simulink model "sim_new_traj_only_att_ctrl"  (R2020a)
settings: Solver=ode4  StartTime=0.0  StopTime=30.0  FixedStep=0.01  RelTol=1e-3
values from neighbouring files (symbols this model uses):
  beta_Phi_1 = pp0 * cal_frac_squ( 3, p_p0_plus_1, q_p0_plus_1 )                          * cal_frac_squ( eps_s_bar / pi, p_p0_min_2, q_p0_min_2 )                          / ( 2 * ( 2 * pp0 - 1 ) * tanh( gamma0 * ( eps_s_bar / pi ) / 2 ) )                          - ( cal_frac_squ( 3, p_p0_plus_1, q_p0_plus_1 ) * gamma0 / ( 4 * ( 2 * pp0 -1 ) ) )                          * cal_frac_squ( eps_s_bar / pi, p_p0_min_ ...(+136 chars)    [init_new_traj_only_att_ctrl.m]
  beta_Phi_2 = ( 1 - pp0 ) * cal_frac_squ( 3, p_p0_plus_1, q_p0_plus_1 )                          / ( 2 * ( 1 - 2 * pp0 ) * cal_frac_squ( eps_s_bar / pi, p_p0_0, q_p0_0 ) * tanh( gamma0 * ( eps_s_bar / pi ) / 2 ) )                          - ( cal_frac_squ( 3, p_p0_plus_1, q_p0_plus_1 ) * gamma0 / ( 4 * ( 1 - 2 * pp0 ) ) )                          * cal_frac_squ( eps_s_bar / pi, p_1_min_p0, q_1_min_p0 )          ...(+112 chars)    [init_new_traj_only_att_ctrl.m]
  c1_diff_sigma_bar_w = diag([12; 12; 12])    [init_new_traj_only_att_ctrl.m]
  c1_diff_ui = diag([25; 30; 20])    [init_new_traj_only_att_ctrl.m]
  c2_diff_sigma_bar_w = diag([12; 12; 12])    [init_new_traj_only_att_ctrl.m]
  c2_diff_ui = diag([50; 50; 10])    [init_new_traj_only_att_ctrl.m]
  c3_diff_sigma_bar_w = diag([15; 15; 15])    [init_new_traj_only_att_ctrl.m]
  c3_diff_ui = diag([15; 15; 10])    [init_new_traj_only_att_ctrl.m]
  c_w_1 = diag( [20; 15; 15] )    [init_new_traj_only_att_ctrl.m]
  c_w_2 = diag( [20; 15; 15] )    [init_new_traj_only_att_ctrl.m]
  c_w_3 = diag( [2; 2; 2] )    [init_new_traj_only_att_ctrl.m]
  cS0 = diag( [4.5; 4.5; 4.5] )    [init_new_traj_only_att_ctrl.m]
  dw_aa_t = 0.2 * ones(3, 5) + ( 1.0 - 0.2 ) * rand(3, 5)    [init_new_traj_only_att_ctrl.m]
  dw_ff_t = [ 0.4 * ones(1, 5) + ( 1.0 - 0.4 ) * rand(1, 5);                      0.4 * ones(1, 5) + ( 1.0 - 0.4 ) * rand(1, 5);                      0.2 * ones(1, 5) + ( 0.6 - 0.2 ) * rand(1, 5) ]    [init_new_traj_only_att_ctrl.m]
  dw_phi_t = ( - pi / 2 ) * ones(3, 5) + ( pi / 2 - ( - pi / 2 ) ) * rand(3, 5)    [init_new_traj_only_att_ctrl.m]
  dwci_init = zeros(3,5)    [init_new_traj_only_att_ctrl.m]
  eps_s_bar_div_pi = eps_s_bar / pi    (= 0.03)    [init_new_traj_only_att_ctrl.m]
  gamma0 = 20    [init_new_traj_only_att_ctrl.m]
  h1w = diag([20.0; 20.0; 20.0])    [init_new_traj_only_att_ctrl.m]
  h2w = diag([30.0; 35.0; 35.0])    [init_new_traj_only_att_ctrl.m]
  h3w = diag([30.0; 25.0; 30.0])    [init_new_traj_only_att_ctrl.m]
  Ji = zeros(3,3,NF)    [init_new_traj_only_att_ctrl.m]
  k_J_0 = diag( [1; 1; 1] )    [init_new_traj_only_att_ctrl.m]
  Lamd_diff_sigma_bar_w = 0.8    [init_new_traj_only_att_ctrl.m]
  Lamd_diff_ui = 0.8    [init_new_traj_only_att_ctrl.m]
  mu_c_theta = 100    [init_new_traj_only_att_ctrl.m]
  mu_d_w = 100    [init_new_traj_only_att_ctrl.m]
  pos0 = zeros(3, 1)    [init_new_traj_only_att_ctrl.m]
  pp0 = 8 / 11    (= 0.727272727273)    [init_new_traj_only_att_ctrl.m]
  PZ0 = P0(3)    [init_new_traj_only_att_ctrl.m]
  PZ1 = 10    [init_new_traj_only_att_ctrl.m]
  Qci_init = repmat([1;0;0;0],1,NF)    [init_new_traj_only_att_ctrl.m]
  R0 = 4    [init_new_traj_only_att_ctrl.m]
  R1 = 8    [init_new_traj_only_att_ctrl.m]
  Rci_init = zeros(3,3,NF)    [init_new_traj_only_att_ctrl.m]
  Ri_init = zeros(3,3,NF)    [init_new_traj_only_att_ctrl.m]
  Rx2 = 10    [init_new_traj_only_att_ctrl.m]
  Ry2 = 6    [init_new_traj_only_att_ctrl.m]
  Rz2 = 4    [init_new_traj_only_att_ctrl.m]
  T0 = 0    [init_new_traj_only_att_ctrl.m]
  T1 = tseq1    (= 10)    [init_new_traj_only_att_ctrl.m]
  T2 = tseq1 + tseq12 + tseq2    (= 30)    [init_new_traj_only_att_ctrl.m]
  thr_p_plus_1 = cal_frac_squ( 3, p_p0_plus_1, q_p0_plus_1 )    [init_new_traj_only_att_ctrl.m]
  ui_init = zeros(3,NF)    [init_new_traj_only_att_ctrl.m]
  vel0 = zeros(3, 1)    [init_new_traj_only_att_ctrl.m]
  wci_init = zeros(3,5)    [init_new_traj_only_att_ctrl.m]
  zeta_diff_sigma_bar_w = 0.3    [init_new_traj_only_att_ctrl.m]
  zeta_diff_ui = 0.05    [init_new_traj_only_att_ctrl.m]
undefined symbols (not defined in the file or in its folder): cal_frac_squ, p_2_p0, p_alfaw1, p_alfaw2, p_beta_w_1, p_beta_w_2, p_p0_min_1, p_p0_plus_1, q_2_p0, q_alfaw1, q_alfaw2, q_beta_w_1, q_beta_w_2, q_p0_min_1, q_p0_plus_1, Qei_init, Qi_init, Rei_init, V_Phi_Rei_init, wei_init, wi_init
(part 3 of 5)

== matlab function sim_new_traj_only_att_ctrl/cal differentiator d_sigma_bar_w_hat agent 3/trans to column23 ==
  data: x input; y output
function y = fcn(x)
y = x(:);

== matlab function sim_new_traj_only_att_ctrl/cal differentiator d_sigma_bar_w_hat agent 3/trans to column24 ==
  data: x input; y output
function y = fcn(x)
y = x(:);

== matlab function sim_new_traj_only_att_ctrl/cal differentiator d_sigma_bar_w_hat agent 3/trans to column25 ==
  data: x input; y output
function y = fcn(x)
y = x(:);

== matlab function sim_new_traj_only_att_ctrl/cal differentiator d_sigma_bar_w_hat agent 4/cal differentiator ==
  data: c1 input; d_sigma_bar_v_hat output; d_dsigma_bar_v_hat output; d_d2sigma_bar_v_hat output; c2 input; c3 input; chi_t input; sigma_bar_v_sig_1 input; sigma_bar_v_sig_2 input; sigma_bar_v_sig_3 input; sigma_bar_v_sig_4 input; sigma_bar_v_sig_5 input; sigma_bar_v_sig_6 input; d_sigma_bar_v_hat input; d2_sigma_bar_v_hat input
function [d_sigma_bar_v_hat, d_dsigma_bar_v_hat, d_d2sigma_bar_v_hat] = fcn(c1, c2, c3, chi_t, sigma_bar_v_sig_1, sigma_bar_v_sig_2, sigma_bar_v_sig_3, ...
                                                                                                                                                sigma_bar_v_sig_4, sigma_bar_v_sig_5, sigma_bar_v_sig_6, d_sigma_bar_v_hat, d2_sigma_bar_v_hat)
d_d2sigma_bar_v_hat = -chi_t .* c1 * sigma_bar_v_sig_1(:) - (1 - chi_t) .* c1 * sigma_bar_v_sig_2(:);
d_dsigma_bar_v_hat = -chi_t .* c2 * sigma_bar_v_sig_3(:) - (1 - chi_t) .* c2 * sigma_bar_v_sig_4(:) + d2_sigma_bar_v_hat(:);
d_sigma_bar_v_hat = -chi_t .* c3 * sigma_bar_v_sig_5(:) - (1 - chi_t) .* c3 * sigma_bar_v_sig_6(:) + d_sigma_bar_v_hat(:);

== matlab function sim_new_traj_only_att_ctrl/cal differentiator d_sigma_bar_w_hat agent 4/cal sig ==
  data: x input; z output; y input
function z = fcn(x, y)
z = x(:) .* sign(y(:));

== matlab function sim_new_traj_only_att_ctrl/cal differentiator d_sigma_bar_w_hat agent 4/cal sig1 ==
  data: x input; z output; y input
function z = fcn(x, y)
z = x(:) .* sign(y(:));

== matlab function sim_new_traj_only_att_ctrl/cal differentiator d_sigma_bar_w_hat agent 4/cal sig2 ==
  data: x input; z output; y input
function z = fcn(x, y)
z = x(:) .* sign(y(:));

== matlab function sim_new_traj_only_att_ctrl/cal differentiator d_sigma_bar_w_hat agent 4/cal sig3 ==
  data: x input; z output; y input
function z = fcn(x, y)
z = x(:) .* sign(y(:));

== matlab function sim_new_traj_only_att_ctrl/Qei dynam agent 5 ==
  data: Qei_vec input; dQei_5 output; wei_vec input
function dQei_5 = fcn(Qei_vec, wei_vec)
%%%% 更新四元数误差微分方程
iiuav = 5;

wei = wei_vec(:,iiuav);
thetaei = Qei_vec(1,iiuav);
qei = Qei_vec(2:4,iiuav);

GammaQei = zeros(4,3);
GammaQei(1,:) = -(qei');
GammaQei(2:4,:) = thetaei*eye(3,3) + cal_askew_mat(qei);
dQei_5 = (1/2)*GammaQei*wei;

end

== matlab function sim_new_traj_only_att_ctrl/cal differentiator d_sigma_bar_w_hat agent 4/cal sig4 ==
  data: x input; z output; y input
function z = fcn(x, y)
z = x(:) .* sign(y(:));

== matlab function sim_new_traj_only_att_ctrl/cal differentiator d_sigma_bar_w_hat agent 4/cal sig5 ==
  data: x input; z output; y input
function z = fcn(x, y)
z = x(:) .* sign(y(:));

== matlab function sim_new_traj_only_att_ctrl/cal differentiator d_sigma_bar_w_hat agent 4/choose sigma_bar_w ==
  data: x input; y output
function y = fcn(x)
iiuav = 4;
y = x(:,iiuav);

== matlab function sim_new_traj_only_att_ctrl/cal differentiator d_sigma_bar_w_hat agent 4/trans to column20 ==
  data: x input; y output
function y = fcn(x)
y = x(:);

== matlab function sim_new_traj_only_att_ctrl/cal differentiator d_sigma_bar_w_hat agent 4/trans to column21 ==
  data: x input; y output
function y = fcn(x)
y = x(:);

== matlab function sim_new_traj_only_att_ctrl/cal differentiator d_sigma_bar_w_hat agent 4/trans to column22 ==
  data: x input; y output
function y = fcn(x)
y = x(:);

== matlab function sim_new_traj_only_att_ctrl/cal differentiator d_sigma_bar_w_hat agent 4/trans to column23 ==
  data: x input; y output
function y = fcn(x)
y = x(:);

== matlab function sim_new_traj_only_att_ctrl/cal differentiator d_sigma_bar_w_hat agent 4/trans to column24 ==
  data: x input; y output
function y = fcn(x)
y = x(:);

== matlab function sim_new_traj_only_att_ctrl/cal differentiator d_sigma_bar_w_hat agent 4/trans to column25 ==
  data: x input; y output
function y = fcn(x)
y = x(:);

== matlab function sim_new_traj_only_att_ctrl/cal differentiator d_sigma_bar_w_hat agent 5/cal differentiator ==
  data: c1 input; d_sigma_bar_v_hat output; d_dsigma_bar_v_hat output; d_d2sigma_bar_v_hat output; c2 input; c3 input; chi_t input; sigma_bar_v_sig_1 input; sigma_bar_v_sig_2 input; sigma_bar_v_sig_3 input; sigma_bar_v_sig_4 input; sigma_bar_v_sig_5 input; sigma_bar_v_sig_6 input; d_sigma_bar_v_hat input; d2_sigma_bar_v_hat input
function [d_sigma_bar_v_hat, d_dsigma_bar_v_hat, d_d2sigma_bar_v_hat] = fcn(c1, c2, c3, chi_t, sigma_bar_v_sig_1, sigma_bar_v_sig_2, sigma_bar_v_sig_3, ...
                                                                                                                                                sigma_bar_v_sig_4, sigma_bar_v_sig_5, sigma_bar_v_sig_6, d_sigma_bar_v_hat, d2_sigma_bar_v_hat)
d_d2sigma_bar_v_hat = -chi_t .* c1 * sigma_bar_v_sig_1(:) - (1 - chi_t) .* c1 * sigma_bar_v_sig_2(:);
d_dsigma_bar_v_hat = -chi_t .* c2 * sigma_bar_v_sig_3(:) - (1 - chi_t) .* c2 * sigma_bar_v_sig_4(:) + d2_sigma_bar_v_hat(:);
d_sigma_bar_v_hat = -chi_t .* c3 * sigma_bar_v_sig_5(:) - (1 - chi_t) .* c3 * sigma_bar_v_sig_6(:) + d_sigma_bar_v_hat(:);

== matlab function sim_new_traj_only_att_ctrl/Qi dynam agent 1 ==
  data: Qi_vec input; dQi_1 output; wi_vec input
function dQi_1 = fcn(Qi_vec, wi_vec)
%%%% 更新四元数微分方程
iiuav = 1;

wi = wi_vec(:,iiuav);
thetai = Qi_vec(1,iiuav);
qi = Qi_vec(2:4,iiuav);

GammaQi = zeros(4,3);
GammaQi(1,:) = -(qi');
GammaQi(2:4,:) = thetai*eye(3,3) + cal_askew_mat(qi);
dQi_1 = (1/2)*GammaQi*wi;

end

== matlab function sim_new_traj_only_att_ctrl/cal differentiator d_sigma_bar_w_hat agent 5/cal sig ==
  data: x input; z output; y input
function z = fcn(x, y)
z = x(:) .* sign(y(:));

== matlab function sim_new_traj_only_att_ctrl/cal differentiator d_sigma_bar_w_hat agent 5/cal sig1 ==
  data: x input; z output; y input
function z = fcn(x, y)
z = x(:) .* sign(y(:));

== matlab function sim_new_traj_only_att_ctrl/cal differentiator d_sigma_bar_w_hat agent 5/cal sig2 ==
  data: x input; z output; y input
function z = fcn(x, y)
z = x(:) .* sign(y(:));

== matlab function sim_new_traj_only_att_ctrl/cal differentiator d_sigma_bar_w_hat agent 5/cal sig3 ==
  data: x input; z output; y input
function z = fcn(x, y)
z = x(:) .* sign(y(:));

== matlab function sim_new_traj_only_att_ctrl/cal differentiator d_sigma_bar_w_hat agent 5/cal sig4 ==
  data: x input; z output; y input
function z = fcn(x, y)
z = x(:) .* sign(y(:));

== matlab function sim_new_traj_only_att_ctrl/cal differentiator d_sigma_bar_w_hat agent 5/cal sig5 ==
  data: x input; z output; y input
function z = fcn(x, y)
z = x(:) .* sign(y(:));

== matlab function sim_new_traj_only_att_ctrl/cal differentiator d_sigma_bar_w_hat agent 5/choose sigma_bar_w ==
  data: x input; y output
function y = fcn(x)
iiuav = 5;
y = x(:,iiuav);

== matlab function sim_new_traj_only_att_ctrl/cal differentiator d_sigma_bar_w_hat agent 5/trans to column20 ==
  data: x input; y output
function y = fcn(x)
y = x(:);

== matlab function sim_new_traj_only_att_ctrl/cal differentiator d_sigma_bar_w_hat agent 5/trans to column21 ==
  data: x input; y output
function y = fcn(x)
y = x(:);

== matlab function sim_new_traj_only_att_ctrl/cal differentiator d_sigma_bar_w_hat agent 5/trans to column22 ==
  data: x input; y output
function y = fcn(x)
y = x(:);

== matlab function sim_new_traj_only_att_ctrl/Qi dynam agent 2 ==
  data: Qi_vec input; dQi_2 output; wi_vec input
function dQi_2 = fcn(Qi_vec, wi_vec)
%%%% 更新四元数微分方程
iiuav = 2;

wi = wi_vec(:,iiuav);
thetai = Qi_vec(1,iiuav);
qi = Qi_vec(2:4,iiuav);

GammaQi = zeros(4,3);
GammaQi(1,:) = -(qi');
GammaQi(2:4,:) = thetai*eye(3,3) + cal_askew_mat(qi);
dQi_2 = (1/2)*GammaQi*wi;

end

== matlab function sim_new_traj_only_att_ctrl/cal differentiator d_sigma_bar_w_hat agent 5/trans to column23 ==
  data: x input; y output
function y = fcn(x)
y = x(:);

== matlab function sim_new_traj_only_att_ctrl/cal differentiator d_sigma_bar_w_hat agent 5/trans to column24 ==
  data: x input; y output
function y = fcn(x)
y = x(:);

== matlab function sim_new_traj_only_att_ctrl/cal differentiator d_sigma_bar_w_hat agent 5/trans to column25 ==
  data: x input; y output
function y = fcn(x)
y = x(:);

== matlab function sim_new_traj_only_att_ctrl/cal divide pi ==
  data: x input; y output
function y = fcn(x)
y = x ./ pi;

== matlab function sim_new_traj_only_att_ctrl/cal dw_hat agent 1 ==
  data: h3w input; Ji input; d_sigma_bar_w_vec input; sigma_bar_w_hat_vec input; dw_hat_1 output
function dw_hat_1 = fcn(h3w, Ji, d_sigma_bar_w_vec, sigma_bar_w_hat_vec)
%%%% 计算扰动观测值dw_hat
iiuav = 1;
dw_hat_1 = Ji(:,:,iiuav) * d_sigma_bar_w_vec(:,iiuav) + h3w * sigma_bar_w_hat_vec(:,iiuav);

== matlab function sim_new_traj_only_att_ctrl/cal dw_hat agent 2 ==
  data: h3w input; Ji input; d_sigma_bar_w_vec input; sigma_bar_w_hat_vec input; dw_hat_2 output
function dw_hat_2 = fcn(h3w, Ji, d_sigma_bar_w_vec, sigma_bar_w_hat_vec)
%%%% 计算扰动观测值dw_hat
iiuav = 2;
dw_hat_2 = Ji(:,:,iiuav) * d_sigma_bar_w_vec(:,iiuav) + h3w * sigma_bar_w_hat_vec(:,iiuav);

== matlab function sim_new_traj_only_att_ctrl/cal dw_hat agent 3 ==
  data: h3w input; Ji input; d_sigma_bar_w_vec input; sigma_bar_w_hat_vec input; dw_hat_3 output
function dw_hat_3 = fcn(h3w, Ji, d_sigma_bar_w_vec, sigma_bar_w_hat_vec)
%%%% 计算扰动观测值dw_hat
iiuav = 3;
dw_hat_3 = Ji(:,:,iiuav) * d_sigma_bar_w_vec(:,iiuav) + h3w * sigma_bar_w_hat_vec(:,iiuav);

== matlab function sim_new_traj_only_att_ctrl/cal dw_hat agent 4 ==
  data: h3w input; Ji input; d_sigma_bar_w_vec input; sigma_bar_w_hat_vec input; dw_hat_4 output
function dw_hat_4 = fcn(h3w, Ji, d_sigma_bar_w_vec, sigma_bar_w_hat_vec)
%%%% 计算扰动观测值dw_hat
iiuav = 4;
dw_hat_4 = Ji(:,:,iiuav) * d_sigma_bar_w_vec(:,iiuav) + h3w * sigma_bar_w_hat_vec(:,iiuav);

== matlab function sim_new_traj_only_att_ctrl/cal dw_hat agent 5 ==
  data: h3w input; Ji input; d_sigma_bar_w_vec input; sigma_bar_w_hat_vec input; dw_hat_5 output
function dw_hat_5 = fcn(h3w, Ji, d_sigma_bar_w_vec, sigma_bar_w_hat_vec)
%%%% 计算扰动观测值dw_hat
iiuav = 5;
dw_hat_5 = Ji(:,:,iiuav) * d_sigma_bar_w_vec(:,iiuav) + h3w * sigma_bar_w_hat_vec(:,iiuav);

== matlab function sim_new_traj_only_att_ctrl/Qi dynam agent 3 ==
  data: Qi_vec input; dQi_3 output; wi_vec input
function dQi_3 = fcn(Qi_vec, wi_vec)
%%%% 更新四元数微分方程
iiuav = 3;

wi = wi_vec(:,iiuav);
thetai = Qi_vec(1,iiuav);
qi = Qi_vec(2:4,iiuav);

GammaQi = zeros(4,3);
GammaQi(1,:) = -(qi');
GammaQi(2:4,:) = thetai*eye(3,3) + cal_askew_mat(qi);
dQi_3 = (1/2)*GammaQi*wi;

end

== matlab function sim_new_traj_only_att_ctrl/cal error dw_tilt ==
  data: dw_vec input; dw_hat_vec input; dw_tilt_vec output
function dw_tilt_vec = fcn(dw_vec, dw_hat_vec)
%%%% 计算扰动观测误差dw_tilt
dw_tilt_vec = zeros(3,5);
for iiuav = 1:5
    dw_tilt_vec(:,iiuav) = dw_vec(:,iiuav) - dw_hat_vec(:,iiuav);
end

== matlab function sim_new_traj_only_att_ctrl/cal sig ==
  data: x input; z output; y input
function z = fcn(x, y)
z = x(:) .* sign(y(:));

== matlab function sim_new_traj_only_att_ctrl/cal sig1 ==
  data: x input; z output; y input
function z = fcn(x, y)
z = x(:) .* sign(y(:));

== matlab function sim_new_traj_only_att_ctrl/cal sig10 ==
  data: x input; z output; y input
function z = fcn(x, y)
z = x(:) .* sign(y(:));

== matlab function sim_new_traj_only_att_ctrl/cal sig11 ==
  data: x input; z output; y input
function z = fcn(x, y)
z = x(:) .* sign(y(:));

== matlab function sim_new_traj_only_att_ctrl/cal sig12 ==
  data: x input; z output; y input
function z = fcn(x, y)
z = x(:) .* sign(y(:));

== matlab function sim_new_traj_only_att_ctrl/cal sig13 ==
  data: x input; z output; y input
function z = fcn(x, y)
z = x(:) .* sign(y(:));

== matlab function sim_new_traj_only_att_ctrl/cal sig14 ==
  data: x input; z output; y input
function z = fcn(x, y)
z = x(:) .* sign(y(:));

== matlab function sim_new_traj_only_att_ctrl/cal sig15 ==
  data: x input; z output; y input
function z = fcn(x, y)
z = x(:) .* sign(y(:));

== matlab function sim_new_traj_only_att_ctrl/cal sig16 ==
  data: x input; z output; y input
function z = fcn(x, y)
z = x(:) .* sign(y(:));

== matlab function sim_new_traj_only_att_ctrl/Qi dynam agent 4 ==
  data: Qi_vec input; dQi_4 output; wi_vec input
function dQi_4 = fcn(Qi_vec, wi_vec)
%%%% 更新四元数微分方程
iiuav = 4;

wi = wi_vec(:,iiuav);
thetai = Qi_vec(1,iiuav);
qi = Qi_vec(2:4,iiuav);

GammaQi = zeros(4,3);
GammaQi(1,:) = -(qi');
GammaQi(2:4,:) = thetai*eye(3,3) + cal_askew_mat(qi);
dQi_4 = (1/2)*GammaQi*wi;

end

== matlab function sim_new_traj_only_att_ctrl/cal sig17 ==
  data: x input; z output; y input
function z = fcn(x, y)
z = x(:) .* sign(y(:));

== matlab function sim_new_traj_only_att_ctrl/cal sig18 ==
  data: x input; z output; y input
function z = fcn(x, y)
z = x(:) .* sign(y(:));

== matlab function sim_new_traj_only_att_ctrl/cal sig19 ==
  data: x input; z output; y input
function z = fcn(x, y)
z = x(:) .* sign(y(:));

== matlab function sim_new_traj_only_att_ctrl/cal sig2 ==
  data: x input; z output; y input
function z = fcn(x, y)
z = x(:) .* sign(y(:));

== matlab function sim_new_traj_only_att_ctrl/cal sig20 ==
  data: x input; z output; y input
function z = fcn(x, y)
z = x(:) .* sign(y(:));

== matlab function sim_new_traj_only_att_ctrl/cal sig21 ==
  data: x input; z output; y input
function z = fcn(x, y)
z = x(:) .* sign(y(:));

== matlab function sim_new_traj_only_att_ctrl/cal sig22 ==
  data: x input; z output; y input
function z = fcn(x, y)
z = x(:) .* sign(y(:));

== matlab function sim_new_traj_only_att_ctrl/cal sig23 ==
  data: x input; z output; y input
function z = fcn(x, y)
z = x(:) .* sign(y(:));

== matlab function sim_new_traj_only_att_ctrl/cal sig24 ==
  data: x input; z output; y input
function z = fcn(x, y)
z = x(:) .* sign(y(:));

== matlab function sim_new_traj_only_att_ctrl/cal sig25 ==
  data: x input; z output; y input
function z = fcn(x, y)
z = x(:) .* sign(y(:));

== matlab function sim_new_traj_only_att_ctrl/Qi dynam agent 5 ==
  data: Qi_vec input; dQi_5 output; wi_vec input
function dQi_5 = fcn(Qi_vec, wi_vec)
%%%% 更新四元数微分方程
iiuav = 5;

wi = wi_vec(:,iiuav);
thetai = Qi_vec(1,iiuav);
qi = Qi_vec(2:4,iiuav);

GammaQi = zeros(4,3);
GammaQi(1,:) = -(qi');
GammaQi(2:4,:) = thetai*eye(3,3) + cal_askew_mat(qi);
dQi_5 = (1/2)*GammaQi*wi;

end

== matlab function sim_new_traj_only_att_ctrl/cal sig26 ==
  data: x input; z output; y input
function z = fcn(x, y)
z = x(:) .* sign(y(:));

== matlab function sim_new_traj_only_att_ctrl/cal sig27 ==
  data: x input; z output; y input
function z = fcn(x, y)
z = x(:) .* sign(y(:));

== matlab function sim_new_traj_only_att_ctrl/cal sig28 ==
  data: x input; z output; y input
function z = fcn(x, y)
z = x(:) .* sign(y(:));

== matlab function sim_new_traj_only_att_ctrl/cal sig29 ==
  data: x input; z output; y input
function z = fcn(x, y)
z = x(:) .* sign(y(:));

== matlab function sim_new_traj_only_att_ctrl/cal sig3 ==
  data: x input; z output; y input
function z = fcn(x, y)
z = x(:) .* sign(y(:));

== matlab function sim_new_traj_only_att_ctrl/cal sig4 ==
  data: x input; z output; y input
function z = fcn(x, y)
z = x(:) .* sign(y(:));

== matlab function sim_new_traj_only_att_ctrl/cal sig5 ==
  data: x input; z output; y input
function z = fcn(x, y)
z = x(:) .* sign(y(:));

== matlab function sim_new_traj_only_att_ctrl/cal sig6 ==
  data: x input; z output; y input
function z = fcn(x, y)
z = x(:) .* sign(y(:));

== matlab function sim_new_traj_only_att_ctrl/cal sig7 ==
  data: x input; z output; y input
function z = fcn(x, y)
z = x(:) .* sign(y(:));

== matlab function sim_new_traj_only_att_ctrl/cal sig8 ==
  data: x input; z output; y input
function z = fcn(x, y)
z = x(:) .* sign(y(:));

== matlab function sim_new_traj_only_att_ctrl/cal Fi_S agent 1 ==
  data: cS0 input; Ji input; wi_vec input; wci_vec input; wei_vec input; Fi_S_1 output; dwci_vec input; Rei_vec input; Phi_bar_psi_e_vec input
function Fi_S_1 = fcn(cS0, Ji, wi_vec, wci_vec, wei_vec, dwci_vec, Rei_vec, Phi_bar_psi_e_vec)
%%%% 计算补偿项
iiuav = 1;
Fi_S_1 = -cal_askew_mat( wi_vec(:,iiuav) ) * Ji(:,:,iiuav) * wi_vec(:,iiuav) ...
                + Ji(:,:,iiuav) * cal_askew_mat( wei_vec(:,iiuav) ) * ( Rei_vec(:,:,iiuav)' ) * wci_vec(:,iiuav) ...
                - Ji(:,:,iiuav) * ( Rei_vec(:,:,iiuav)' ) * dwci_vec(:,iiuav) ...
                + cS0 * Ji(:,:,iiuav) * Phi_bar_psi_e_vec(:,iiuav);

== matlab function sim_new_traj_only_att_ctrl/cal sig9 ==
  data: x input; z output; y input
function z = fcn(x, y)
z = x(:) .* sign(y(:));

== matlab function sim_new_traj_only_att_ctrl/cal sigma_bar_w_hat agent 1 ==
  data: h1w input; h2w input; theta_sigma_bar_w_tilt_1_vec input; d_sigma_bar_w_hat_1 output; theta_sigma_bar_w_tilt_2_vec input; d_sigma_bar_w_vec input
function d_sigma_bar_w_hat_1 = fcn(h1w, h2w, theta_sigma_bar_w_tilt_1_vec, theta_sigma_bar_w_tilt_2_vec, d_sigma_bar_w_vec)
%%%% 计算扰动观测器中虚拟速度控制量观测值sigma_w_hat的微分方程
iiuav = 1;
d_sigma_bar_w_hat_1 = d_sigma_bar_w_vec(:,iiuav) + ...
                                            h1w * theta_sigma_bar_w_tilt_1_vec(:,iiuav) + ...
                                            h2w * theta_sigma_bar_w_tilt_2_vec(:,iiuav);

== matlab function sim_new_traj_only_att_ctrl/cal sigma_bar_w_hat agent 2 ==
  data: h1w input; h2w input; theta_sigma_bar_w_tilt_1_vec input; d_sigma_bar_w_hat_2 output; theta_sigma_bar_w_tilt_2_vec input; d_sigma_bar_w_vec input
function d_sigma_bar_w_hat_2 = fcn(h1w, h2w, theta_sigma_bar_w_tilt_1_vec, theta_sigma_bar_w_tilt_2_vec, d_sigma_bar_w_vec)
%%%% 计算扰动观测器中虚拟速度控制量观测值sigma_v_hat的微分方程
iiuav = 2;
d_sigma_bar_w_hat_2 = d_sigma_bar_w_vec(:,iiuav) + ...
                                            h1w * theta_sigma_bar_w_tilt_1_vec(:,iiuav) + ...
                                            h2w * theta_sigma_bar_w_tilt_2_vec(:,iiuav);

== matlab function sim_new_traj_only_att_ctrl/cal sigma_bar_w_hat agent 3 ==
  data: h1w input; h2w input; theta_sigma_bar_w_tilt_1_vec input; d_sigma_bar_w_hat_3 output; theta_sigma_bar_w_tilt_2_vec input; d_sigma_bar_w_vec input
function d_sigma_bar_w_hat_3 = fcn(h1w, h2w, theta_sigma_bar_w_tilt_1_vec, theta_sigma_bar_w_tilt_2_vec, d_sigma_bar_w_vec)
%%%% 计算扰动观测器中虚拟速度控制量观测值sigma_w_hat的微分方程
iiuav = 3;
d_sigma_bar_w_hat_3 = d_sigma_bar_w_vec(:,iiuav) + ...
                                            h1w * theta_sigma_bar_w_tilt_1_vec(:,iiuav) + ...
                                            h2w * theta_sigma_bar_w_tilt_2_vec(:,iiuav);

== matlab function sim_new_traj_only_att_ctrl/cal sigma_bar_w_hat agent 4 ==
  data: h1w input; h2w input; theta_sigma_bar_w_tilt_1_vec input; d_sigma_bar_w_hat_4 output; theta_sigma_bar_w_tilt_2_vec input; d_sigma_bar_w_vec input
function d_sigma_bar_w_hat_4 = fcn(h1w, h2w, theta_sigma_bar_w_tilt_1_vec, theta_sigma_bar_w_tilt_2_vec, d_sigma_bar_w_vec)
%%%% 计算扰动观测器中虚拟速度控制量观测值sigma_w_hat的微分方程
iiuav = 4;
d_sigma_bar_w_hat_4 = d_sigma_bar_w_vec(:,iiuav) + ...
                                            h1w * theta_sigma_bar_w_tilt_1_vec(:,iiuav) + ...
                                            h2w * theta_sigma_bar_w_tilt_2_vec(:,iiuav);

== matlab function sim_new_traj_only_att_ctrl/cal sigma_bar_w_hat agent 5 ==
  data: h1w input; h2w input; theta_sigma_bar_w_tilt_1_vec input; d_sigma_bar_w_hat_5 output; theta_sigma_bar_w_tilt_2_vec input; d_sigma_bar_w_vec input
function d_sigma_bar_w_hat_5 = fcn(h1w, h2w, theta_sigma_bar_w_tilt_1_vec, theta_sigma_bar_w_tilt_2_vec, d_sigma_bar_w_vec)
%%%% 计算扰动观测器中虚拟速度控制量观测值sigma_w_hat的微分方程
iiuav = 5;
d_sigma_bar_w_hat_5 = d_sigma_bar_w_vec(:,iiuav) + ...
                                            h1w * theta_sigma_bar_w_tilt_1_vec(:,iiuav) + ...
                                            h2w * theta_sigma_bar_w_tilt_2_vec(:,iiuav);

== matlab function sim_new_traj_only_att_ctrl/cal sigma_w_bar ==
  data: sigma_bar_w_vec output; wi_vec input; sigma_w_vec input
function sigma_bar_w_vec = fcn(wi_vec, sigma_w_vec)
%%%% 计算姿态角速率跟踪误差
sigma_bar_w_vec = zeros(3,5);
for iiuav = 1:5
    sigma_bar_w_vec(:,iiuav) = wi_vec(:,iiuav) - sigma_w_vec(:,iiuav);
end

== matlab function sim_new_traj_only_att_ctrl/cal taui agent 1 ==
  data: c_w_1 input; c_w_2 input; c_w_3 input; k_J_0 input; tau_1 output; Ji input; Si_vec input; dw_hat_vec input; Fi_S_vec input; theta_Si_beta_w_1_vec input; theta_Si_beta_w_2_vec input
function tau_1 = fcn(c_w_1, c_w_2, c_w_3, k_J_0, Ji, Si_vec, dw_hat_vec, ...
                                        Fi_S_vec, theta_Si_beta_w_1_vec, theta_Si_beta_w_2_vec)
%%%% 计算用于姿态控制的驱动力矩控制输入
iiuav = 1;
tau_1 = -c_w_1 * theta_Si_beta_w_1_vec(:,iiuav) - c_w_2 * theta_Si_beta_w_2_vec(:,iiuav) - c_w_3 * Si_vec(:,iiuav) ...
                - dw_hat_vec(:,iiuav) - k_J_0 * inv( Ji(:,:,iiuav) ) * Fi_S_vec(:,iiuav);
end

== matlab function sim_new_traj_only_att_ctrl/cal taui agent 2 ==
  data: c_w_1 input; c_w_2 input; c_w_3 input; k_J_0 input; tau_2 output; Ji input; Si_vec input; dw_hat_vec input; Fi_S_vec input; theta_Si_beta_w_1_vec input; theta_Si_beta_w_2_vec input
function tau_2 = fcn(c_w_1, c_w_2, c_w_3, k_J_0, Ji, Si_vec, dw_hat_vec, ...
                                        Fi_S_vec, theta_Si_beta_w_1_vec, theta_Si_beta_w_2_vec)
%%%% 计算用于姿态控制的驱动力矩控制输入
iiuav = 2;
tau_2 = -c_w_1 * theta_Si_beta_w_1_vec(:,iiuav) - c_w_2 * theta_Si_beta_w_2_vec(:,iiuav) - c_w_3 * Si_vec(:,iiuav) ...
                - dw_hat_vec(:,iiuav) - k_J_0 * inv( Ji(:,:,iiuav) ) * Fi_S_vec(:,iiuav);
end

== matlab function sim_new_traj_only_att_ctrl/cal taui agent 3 ==
  data: c_w_1 input; c_w_2 input; c_w_3 input; k_J_0 input; tau_3 output; Ji input; Si_vec input; dw_hat_vec input; Fi_S_vec input; theta_Si_beta_w_1_vec input; theta_Si_beta_w_2_vec input
function tau_3 = fcn(c_w_1, c_w_2, c_w_3, k_J_0, Ji, Si_vec, dw_hat_vec, ...
                                        Fi_S_vec, theta_Si_beta_w_1_vec, theta_Si_beta_w_2_vec)
%%%% 计算用于姿态控制的驱动力矩控制输入
iiuav = 3;
tau_3 = -c_w_1 * theta_Si_beta_w_1_vec(:,iiuav) - c_w_2 * theta_Si_beta_w_2_vec(:,iiuav) - c_w_3 * Si_vec(:,iiuav) ...
                - dw_hat_vec(:,iiuav) - k_J_0 * inv( Ji(:,:,iiuav) ) * Fi_S_vec(:,iiuav);
end

== matlab function sim_new_traj_only_att_ctrl/cal taui agent 4 ==
  data: c_w_1 input; c_w_2 input; c_w_3 input; k_J_0 input; tau_4 output; Ji input; Si_vec input; dw_hat_vec input; Fi_S_vec input; theta_Si_beta_w_1_vec input; theta_Si_beta_w_2_vec input
function tau_4 = fcn(c_w_1, c_w_2, c_w_3, k_J_0, Ji, Si_vec, dw_hat_vec, ...
                                        Fi_S_vec, theta_Si_beta_w_1_vec, theta_Si_beta_w_2_vec)
%%%% 计算用于姿态控制的驱动力矩控制输入
iiuav = 4;
tau_4 = -c_w_1 * theta_Si_beta_w_1_vec(:,iiuav) - c_w_2 * theta_Si_beta_w_2_vec(:,iiuav) - c_w_3 * Si_vec(:,iiuav) ...
                - dw_hat_vec(:,iiuav) - k_J_0 * inv( Ji(:,:,iiuav) ) * Fi_S_vec(:,iiuav);
end

== matlab function sim_new_traj_only_att_ctrl/cal taui agent 5 ==
  data: c_w_1 input; c_w_2 input; c_w_3 input; k_J_0 input; tau_5 output; Ji input; Si_vec input; dw_hat_vec input; Fi_S_vec input; theta_Si_beta_w_1_vec input; theta_Si_beta_w_2_vec input
function tau_5 = fcn(c_w_1, c_w_2, c_w_3, k_J_0, Ji, Si_vec, dw_hat_vec, ...
                                        Fi_S_vec, theta_Si_beta_w_1_vec, theta_Si_beta_w_2_vec)
%%%% 计算用于姿态控制的驱动力矩控制输入
iiuav = 5;
tau_5 = -c_w_1 * theta_Si_beta_w_1_vec(:,iiuav) - c_w_2 * theta_Si_beta_w_2_vec(:,iiuav) - c_w_3 * Si_vec(:,iiuav) ...
                - dw_hat_vec(:,iiuav) - k_J_0 * inv( Ji(:,:,iiuav) ) * Fi_S_vec(:,iiuav);
end

== matlab function sim_new_traj_only_att_ctrl/cal Fi_S agent 2 ==
  data: cS0 input; Ji input; wi_vec input; wci_vec input; wei_vec input; Fi_S_2 output; dwci_vec input; Rei_vec input; Phi_bar_psi_e_vec input
function Fi_S_2 = fcn(cS0, Ji, wi_vec, wci_vec, wei_vec, dwci_vec, Rei_vec, Phi_bar_psi_e_vec)
%%%% 计算补偿项
iiuav = 2;
Fi_S_2 = -cal_askew_mat( wi_vec(:,iiuav) ) * Ji(:,:,iiuav) * wi_vec(:,iiuav) ...
                + Ji(:,:,iiuav) * cal_askew_mat( wei_vec(:,iiuav) ) * ( Rei_vec(:,:,iiuav)' ) * wci_vec(:,iiuav) ...
                - Ji(:,:,iiuav) * ( Rei_vec(:,:,iiuav)' ) * dwci_vec(:,iiuav) ...
                + cS0 * Ji(:,:,iiuav) * Phi_bar_psi_e_vec(:,iiuav);

== matlab function sim_new_traj_only_att_ctrl/cal theta_Si_beta_w agent 1 ==
  data: mu_c_theta input; Si_squ_beta_w_1_vec input; theta_Si_beta_w_1_node_1 output; Si_squ_beta_w_2_vec input; Si_vec input; theta_Si_beta_w_2_node_1 output
function [theta_Si_beta_w_1_node_1, theta_Si_beta_w_2_node_1] = fcn(mu_c_theta, Si_squ_beta_w_1_vec, Si_squ_beta_w_2_vec, Si_vec)
%%%% 计算平滑递增函数
iiuav = 1;
theta_Si_beta_w_1_node_1 = Si_squ_beta_w_1_vec(:, iiuav) .* ( -1 + 2 ./ ( 1 + exp( -mu_c_theta .* Si_vec(:,iiuav) ) ) );
theta_Si_beta_w_2_node_1 = Si_squ_beta_w_2_vec(:, iiuav) .* ( -1 + 2 ./ ( 1 + exp( -mu_c_theta .* Si_vec(:,iiuav) ) ) );

== matlab function sim_new_traj_only_att_ctrl/cal theta_Si_beta_w agent 2 ==
  data: mu_c_theta input; Si_squ_beta_w_1_vec input; theta_Si_beta_w_1_node_2 output; Si_squ_beta_w_2_vec input; Si_vec input; theta_Si_beta_w_2_node_2 output
function [theta_Si_beta_w_1_node_2, theta_Si_beta_w_2_node_2] = fcn(mu_c_theta, Si_squ_beta_w_1_vec, Si_squ_beta_w_2_vec, Si_vec)
%%%% 计算平滑递增函数
iiuav = 2;
theta_Si_beta_w_1_node_2 = Si_squ_beta_w_1_vec(:, iiuav) .* ( -1 + 2 ./ ( 1 + exp( -mu_c_theta .* Si_vec(:,iiuav) ) ) );
theta_Si_beta_w_2_node_2 = Si_squ_beta_w_2_vec(:, iiuav) .* ( -1 + 2 ./ ( 1 + exp( -mu_c_theta .* Si_vec(:,iiuav) ) ) );

== matlab function sim_new_traj_only_att_ctrl/cal theta_Si_beta_w agent 3 ==
  data: mu_c_theta input; Si_squ_beta_w_1_vec input; theta_Si_beta_w_1_node_3 output; Si_squ_beta_w_2_vec input; Si_vec input; theta_Si_beta_w_2_node_3 output
function [theta_Si_beta_w_1_node_3, theta_Si_beta_w_2_node_3] = fcn(mu_c_theta, Si_squ_beta_w_1_vec, Si_squ_beta_w_2_vec, Si_vec)
%%%% 计算平滑递增函数
iiuav = 3;
theta_Si_beta_w_1_node_3 = Si_squ_beta_w_1_vec(:, iiuav) .* ( -1 + 2 ./ ( 1 + exp( -mu_c_theta .* Si_vec(:,iiuav) ) ) );
theta_Si_beta_w_2_node_3 = Si_squ_beta_w_2_vec(:, iiuav) .* ( -1 + 2 ./ ( 1 + exp( -mu_c_theta .* Si_vec(:,iiuav) ) ) );

== matlab function sim_new_traj_only_att_ctrl/cal theta_Si_beta_w agent 4 ==
  data: mu_c_theta input; Si_squ_beta_w_1_vec input; theta_Si_beta_w_1_node_4 output; Si_squ_beta_w_2_vec input; Si_vec input; theta_Si_beta_w_2_node_4 output
function [theta_Si_beta_w_1_node_4, theta_Si_beta_w_2_node_4] = fcn(mu_c_theta, Si_squ_beta_w_1_vec, Si_squ_beta_w_2_vec, Si_vec)
%%%% 计算平滑递增函数
iiuav = 4;
theta_Si_beta_w_1_node_4 = Si_squ_beta_w_1_vec(:, iiuav) .* ( -1 + 2 ./ ( 1 + exp( -mu_c_theta .* Si_vec(:,iiuav) ) ) );
theta_Si_beta_w_2_node_4 = Si_squ_beta_w_2_vec(:, iiuav) .* ( -1 + 2 ./ ( 1 + exp( -mu_c_theta .* Si_vec(:,iiuav) ) ) );

== matlab function sim_new_traj_only_att_ctrl/cal theta_Si_beta_w agent 5 ==
  data: mu_c_theta input; Si_squ_beta_w_1_vec input; theta_Si_beta_w_1_node_5 output; Si_squ_beta_w_2_vec input; Si_vec input; theta_Si_beta_w_2_node_5 output
function [theta_Si_beta_w_1_node_5, theta_Si_beta_w_2_node_5] = fcn(mu_c_theta, Si_squ_beta_w_1_vec, Si_squ_beta_w_2_vec, Si_vec)
%%%% 计算平滑递增函数
iiuav = 5;
theta_Si_beta_w_1_node_5 = Si_squ_beta_w_1_vec(:, iiuav) .* ( -1 + 2 ./ ( 1 + exp( -mu_c_theta .* Si_vec(:,iiuav) ) ) );
theta_Si_beta_w_2_node_5 = Si_squ_beta_w_2_vec(:, iiuav) .* ( -1 + 2 ./ ( 1 + exp( -mu_c_theta .* Si_vec(:,iiuav) ) ) );

== matlab function sim_new_traj_only_att_ctrl/cal theta_sigma_bar_w_tilt agent 1 ==
  data: alfa_theta_obs_w input; sigma_bar_w_tilt_squ_1_1 input; theta_sigma_bar_w_tilt_1_1 output; sigma_bar_w_tilt_squ_2_1 input; sigma_bar_w_tilt_vec input; theta_sigma_bar_w_tilt_2_1 output
function [theta_sigma_bar_w_tilt_1_1, theta_sigma_bar_w_tilt_2_1] = fcn(alfa_theta_obs_w, sigma_bar_w_tilt_squ_1_1, sigma_bar_w_tilt_squ_2_1, sigma_bar_w_tilt_vec)
%%%% 计算平滑递增函数
iiuav = 1;
theta_sigma_bar_w_tilt_1_1 = sigma_bar_w_tilt_squ_1_1(:) .* ( -1 + 2 ./ ( 1 + exp( -alfa_theta_obs_w .* sigma_bar_w_tilt_vec(:,iiuav) ) ) );
theta_sigma_bar_w_tilt_2_1 = sigma_bar_w_tilt_squ_2_1(:) .* ( -1 + 2 ./ ( 1 + exp( -alfa_theta_obs_w .* sigma_bar_w_tilt_vec(:,iiuav) ) ) );

== matlab function sim_new_traj_only_att_ctrl/cal theta_sigma_bar_w_tilt agent 2 ==
  data: alfa_theta_obs_w input; sigma_bar_w_tilt_squ_1_2 input; theta_sigma_bar_w_tilt_1_2 output; sigma_bar_w_tilt_squ_2_2 input; sigma_bar_w_tilt_vec input; theta_sigma_bar_w_tilt_2_2 output
function [theta_sigma_bar_w_tilt_1_2, theta_sigma_bar_w_tilt_2_2] = fcn(alfa_theta_obs_w, sigma_bar_w_tilt_squ_1_2, sigma_bar_w_tilt_squ_2_2, sigma_bar_w_tilt_vec)
%%%% 计算平滑递增函数
iiuav = 2;
theta_sigma_bar_w_tilt_1_2 = sigma_bar_w_tilt_squ_1_2(:) .* ( -1 + 2 ./ ( 1 + exp( -alfa_theta_obs_w .* sigma_bar_w_tilt_vec(:,iiuav) ) ) );
theta_sigma_bar_w_tilt_2_2 = sigma_bar_w_tilt_squ_2_2(:) .* ( -1 + 2 ./ ( 1 + exp( -alfa_theta_obs_w .* sigma_bar_w_tilt_vec(:,iiuav) ) ) );

== matlab function sim_new_traj_only_att_ctrl/cal theta_sigma_bar_w_tilt agent 3 ==
  data: alfa_theta_obs_w input; sigma_bar_w_tilt_squ_1_3 input; theta_sigma_bar_w_tilt_1_3 output; sigma_bar_w_tilt_squ_2_3 input; sigma_bar_w_tilt_vec input; theta_sigma_bar_w_tilt_2_3 output
function [theta_sigma_bar_w_tilt_1_3, theta_sigma_bar_w_tilt_2_3] = fcn(alfa_theta_obs_w, sigma_bar_w_tilt_squ_1_3, sigma_bar_w_tilt_squ_2_3, sigma_bar_w_tilt_vec)
%%%% 计算平滑递增函数
iiuav = 3;
theta_sigma_bar_w_tilt_1_3 = sigma_bar_w_tilt_squ_1_3(:) .* ( -1 + 2 ./ ( 1 + exp( -alfa_theta_obs_w .* sigma_bar_w_tilt_vec(:,iiuav) ) ) );
theta_sigma_bar_w_tilt_2_3 = sigma_bar_w_tilt_squ_2_3(:) .* ( -1 + 2 ./ ( 1 + exp( -alfa_theta_obs_w .* sigma_bar_w_tilt_vec(:,iiuav) ) ) );

== matlab function sim_new_traj_only_att_ctrl/cal theta_sigma_bar_w_tilt agent 4 ==
  data: alfa_theta_obs_w input; sigma_bar_w_tilt_squ_1_4 input; theta_sigma_bar_w_tilt_1_4 output; sigma_bar_w_tilt_squ_2_4 input; sigma_bar_w_tilt_vec input; theta_sigma_bar_w_tilt_2_4 output
function [theta_sigma_bar_w_tilt_1_4, theta_sigma_bar_w_tilt_2_4] = fcn(alfa_theta_obs_w, sigma_bar_w_tilt_squ_1_4, sigma_bar_w_tilt_squ_2_4, sigma_bar_w_tilt_vec)
%%%% 计算平滑递增函数
iiuav = 4;
theta_sigma_bar_w_tilt_1_4 = sigma_bar_w_tilt_squ_1_4(:) .* ( -1 + 2 ./ ( 1 + exp( -alfa_theta_obs_w .* sigma_bar_w_tilt_vec(:,iiuav) ) ) );
theta_sigma_bar_w_tilt_2_4 = sigma_bar_w_tilt_squ_2_4(:) .* ( -1 + 2 ./ ( 1 + exp( -alfa_theta_obs_w .* sigma_bar_w_tilt_vec(:,iiuav) ) ) );

== matlab function sim_new_traj_only_att_ctrl/cal theta_sigma_bar_w_tilt agent 5 ==
  data: alfa_theta_obs_w input; sigma_bar_w_tilt_squ_1_5 input; theta_sigma_bar_w_tilt_1_5 output; sigma_bar_w_tilt_squ_2_5 input; sigma_bar_w_tilt_vec input; theta_sigma_bar_w_tilt_2_5 output
function [theta_sigma_bar_w_tilt_1_5, theta_sigma_bar_w_tilt_2_5] = fcn(alfa_theta_obs_w, sigma_bar_w_tilt_squ_1_5, sigma_bar_w_tilt_squ_2_5, sigma_bar_w_tilt_vec)
%%%% 计算平滑递增函数
iiuav = 5;
theta_sigma_bar_w_tilt_1_5 = sigma_bar_w_tilt_squ_1_5(:) .* ( -1 + 2 ./ ( 1 + exp( -alfa_theta_obs_w .* sigma_bar_w_tilt_vec(:,iiuav) ) ) );
theta_sigma_bar_w_tilt_2_5 = sigma_bar_w_tilt_squ_2_5(:) .* ( -1 + 2 ./ ( 1 + exp( -alfa_theta_obs_w .* sigma_bar_w_tilt_vec(:,iiuav) ) ) );

== matlab function sim_new_traj_only_att_ctrl/cal wci dwci agent 1 ==
  data: ui_vec input; wci output; duihat_vec input; d2uihat_vec input; Rci_mat input; dwci output
function [wci, dwci] = fcn(ui_vec, duihat_vec, d2uihat_vec, Rci_mat)
%%%% 计算姿态角速率指令及其导数

iiuav = 1;
ui = ui_vec(:,iiuav);
duihat = duihat_vec(:,iiuav);
d2uihat = d2uihat_vec(:,iiuav);
Rci = Rci_mat(:,:,iiuav);

ee1 = [1;0;0];
ee2 = [0;1;0];
ee3 = [0;0;1];
RciE3 = ui / norm(ui,2);
PiMat = eye(3,3) - ee3*(ee3');
dRciE3 = (1 / norm(ui,2))*Rci*PiMat*(Rci')*duihat;
Themat = [-RciE3(2)/(1+RciE3(3)),         -RciE3(1)/(1+RciE3(3)),       (RciE3(1)*RciE3(2))/((1+RciE3(3))^2); ...
                   2*RciE3(1)/(1+RciE3(3)),                0,                               1 - (RciE3(1)^2)/((1+RciE3(3))^2); ...
                               0                                       -1                                                        0                                   ];
wcxe3 = (1 / norm(ui,2))*PiMat*(Rci')*duihat;
wcxe2 = (1 / norm(ui,2))*(Rci')*Themat*Rci*PiMat*(Rci')*duihat;
wci = [-wcxe3(2); wcxe3(1); -wcxe2(1)];

TempMat1 = [0,                           -1/(1+RciE3(3)),                   (RciE3(2))/((1+RciE3(3))^2); ...
                       2/(1+RciE3(3)),                0,                               (-2*RciE3(1))/((1+RciE3(3))^2); ...
                       0,                                     0,                                                   0                             ];
TempMat2 = [-1/(1+RciE3(3)),              0,                               (RciE3(1))/((1+RciE3(3))^2); ...
                       0,                                     0,                                                   0                      ; ...
                       0,                                     0,                                                   0                             ];
TempMat3 = [(RciE3(2))/((1+RciE3(3))^2),                 (RciE3(1))/((1+RciE3(3))^2),       (-2*RciE3(1)*RciE3(2))/((1+RciE3(3))^3); ...
                       (-2*RciE3(1))/((1+RciE3(3))^2),                             0,                               (2*(RciE3(1)^2))/((1+RciE3(3))^3); ...
                        0,                                                                          0,                                                   0                             ];
dTheMat = TempMat1*dRciE3*(ee1') + TempMat2*dRciE3*(ee2') + TempMat3*dRciE3*(ee3');
wcix = cal_askew_mat(wci);
dRciT = -wcix*(Rci');
dwcxe3 = (1 / norm(ui,2))*PiMat*(dRciT*duihat+(Rci')*(d2uihat-(((ui')*duihat)/(norm(ui,2)^2))*duihat));
dwcxe2 = (1 / norm(ui,2))*((dRciT*Themat+(Rci')*dTheMat) ...
                *(Rci*PiMat*(Rci'))*duihat + (Rci')*Themat*(Rci*PiMat*(Rci'))*(d2uihat-(((ui')*duihat)/(norm(ui,2)^2))*duihat));
dwci = [-dwcxe3(2);  dwcxe3(1);  -dwcxe2(1)];

== matlab function sim_new_traj_only_att_ctrl/cal wci dwci agent 2 ==
  data: ui_vec input; wci output; duihat_vec input; d2uihat_vec input; Rci_mat input; dwci output
function [wci, dwci] = fcn(ui_vec, duihat_vec, d2uihat_vec, Rci_mat)
%%%% 计算姿态角速率指令及其导数

iiuav = 2;
ui = ui_vec(:,iiuav);
duihat = duihat_vec(:,iiuav);
d2uihat = d2uihat_vec(:,iiuav);
Rci = Rci_mat(:,:,iiuav);

ee1 = [1;0;0];
ee2 = [0;1;0];
ee3 = [0;0;1];
RciE3 = ui / norm(ui,2);
PiMat = eye(3,3) - ee3*(ee3');
dRciE3 = (1 / norm(ui,2))*Rci*PiMat*(Rci')*duihat;
Themat = [-RciE3(2)/(1+RciE3(3)),         -RciE3(1)/(1+RciE3(3)),       (RciE3(1)*RciE3(2))/((1+RciE3(3))^2); ...
                   2*RciE3(1)/(1+RciE3(3)),                0,                               1 - (RciE3(1)^2)/((1+RciE3(3))^2); ...
                               0                                       -1                                                        0                                   ];
wcxe3 = (1 / norm(ui,2))*PiMat*(Rci')*duihat;
wcxe2 = (1 / norm(ui,2))*(Rci')*Themat*Rci*PiMat*(Rci')*duihat;
wci = [-wcxe3(2); wcxe3(1); -wcxe2(1)];

TempMat1 = [0,                           -1/(1+RciE3(3)),                   (RciE3(2))/((1+RciE3(3))^2); ...
                       2/(1+RciE3(3)),                0,                               (-2*RciE3(1))/((1+RciE3(3))^2); ...
                       0,                                     0,                                                   0                             ];
TempMat2 = [-1/(1+RciE3(3)),              0,                               (RciE3(1))/((1+RciE3(3))^2); ...
                       0,                                     0,                                                   0                      ; ...
                       0,                                     0,                                                   0                             ];
TempMat3 = [(RciE3(2))/((1+RciE3(3))^2),                 (RciE3(1))/((1+RciE3(3))^2),       (-2*RciE3(1)*RciE3(2))/((1+RciE3(3))^3); ...
                       (-2*RciE3(1))/((1+RciE3(3))^2),                             0,                               (2*(RciE3(1)^2))/((1+RciE3(3))^3); ...
                        0,                                                                          0,                                                   0                             ];
dTheMat = TempMat1*dRciE3*(ee1') + TempMat2*dRciE3*(ee2') + TempMat3*dRciE3*(ee3');
wcix = cal_askew_mat(wci);
dRciT = -wcix*(Rci');
dwcxe3 = (1 / norm(ui,2))*PiMat*(dRciT*duihat+(Rci')*(d2uihat-(((ui')*duihat)/(norm(ui,2)^2))*duihat));
dwcxe2 = (1 / norm(ui,2))*((dRciT*Themat+(Rci')*dTheMat) ...
                *(Rci*PiMat*(Rci'))*duihat + (Rci')*Themat*(Rci*PiMat*(Rci'))*(d2uihat-(((ui')*duihat)/(norm(ui,2)^2))*duihat));
dwci = [-dwcxe3(2);  dwcxe3(1);  -dwcxe2(1)];

== matlab function sim_new_traj_only_att_ctrl/cal Fi_S agent 3 ==
  data: cS0 input; Ji input; wi_vec input; wci_vec input; wei_vec input; Fi_S_3 output; dwci_vec input; Rei_vec input; Phi_bar_psi_e_vec input
function Fi_S_3 = fcn(cS0, Ji, wi_vec, wci_vec, wei_vec, dwci_vec, Rei_vec, Phi_bar_psi_e_vec)
%%%% 计算补偿项
iiuav = 3;
Fi_S_3 = -cal_askew_mat( wi_vec(:,iiuav) ) * Ji(:,:,iiuav) * wi_vec(:,iiuav) ...
                + Ji(:,:,iiuav) * cal_askew_mat( wei_vec(:,iiuav) ) * ( Rei_vec(:,:,iiuav)' ) * wci_vec(:,iiuav) ...
                - Ji(:,:,iiuav) * ( Rei_vec(:,:,iiuav)' ) * dwci_vec(:,iiuav) ...
                + cS0 * Ji(:,:,iiuav) * Phi_bar_psi_e_vec(:,iiuav);

== matlab function sim_new_traj_only_att_ctrl/cal wci dwci agent 3 ==
  data: ui_vec input; wci output; duihat_vec input; d2uihat_vec input; Rci_mat input; dwci output
function [wci, dwci] = fcn(ui_vec, duihat_vec, d2uihat_vec, Rci_mat)
%%%% 计算姿态角速率指令及其导数

iiuav = 3;
ui = ui_vec(:,iiuav);
duihat = duihat_vec(:,iiuav);
d2uihat = d2uihat_vec(:,iiuav);
Rci = Rci_mat(:,:,iiuav);

ee1 = [1;0;0];
ee2 = [0;1;0];
ee3 = [0;0;1];
RciE3 = ui / norm(ui,2);
PiMat = eye(3,3) - ee3*(ee3');
dRciE3 = (1 / norm(ui,2))*Rci*PiMat*(Rci')*duihat;
Themat = [-RciE3(2)/(1+RciE3(3)),         -RciE3(1)/(1+RciE3(3)),       (RciE3(1)*RciE3(2))/((1+RciE3(3))^2); ...
                   2*RciE3(1)/(1+RciE3(3)),                0,                               1 - (RciE3(1)^2)/((1+RciE3(3))^2); ...
                               0                                       -1                                                        0                                   ];
wcxe3 = (1 / norm(ui,2))*PiMat*(Rci')*duihat;
wcxe2 = (1 / norm(ui,2))*(Rci')*Themat*Rci*PiMat*(Rci')*duihat;
wci = [-wcxe3(2); wcxe3(1); -wcxe2(1)];

TempMat1 = [0,                           -1/(1+RciE3(3)),                   (RciE3(2))/((1+RciE3(3))^2); ...
                       2/(1+RciE3(3)),                0,                               (-2*RciE3(1))/((1+RciE3(3))^2); ...
                       0,                                     0,                                                   0                             ];
TempMat2 = [-1/(1+RciE3(3)),              0,                               (RciE3(1))/((1+RciE3(3))^2); ...
                       0,                                     0,                                                   0                      ; ...
                       0,                                     0,                                                   0                             ];
TempMat3 = [(RciE3(2))/((1+RciE3(3))^2),                 (RciE3(1))/((1+RciE3(3))^2),       (-2*RciE3(1)*RciE3(2))/((1+RciE3(3))^3); ...
                       (-2*RciE3(1))/((1+RciE3(3))^2),                             0,                               (2*(RciE3(1)^2))/((1+RciE3(3))^3); ...
                        0,                                                                          0,                                                   0                             ];
dTheMat = TempMat1*dRciE3*(ee1') + TempMat2*dRciE3*(ee2') + TempMat3*dRciE3*(ee3');
wcix = cal_askew_mat(wci);
dRciT = -wcix*(Rci');
dwcxe3 = (1 / norm(ui,2))*PiMat*(dRciT*duihat+(Rci')*(d2uihat-(((ui')*duihat)/(norm(ui,2)^2))*duihat));
dwcxe2 = (1 / norm(ui,2))*((dRciT*Themat+(Rci')*dTheMat) ...
                *(Rci*PiMat*(Rci'))*duihat + (Rci')*Themat*(Rci*PiMat*(Rci'))*(d2uihat-(((ui')*duihat)/(norm(ui,2)^2))*duihat));
dwci = [-dwcxe3(2);  dwcxe3(1);  -dwcxe2(1)];

== matlab function sim_new_traj_only_att_ctrl/cal wci dwci agent 4 ==
  data: ui_vec input; wci output; duihat_vec input; d2uihat_vec input; Rci_mat input; dwci output
function [wci, dwci] = fcn(ui_vec, duihat_vec, d2uihat_vec, Rci_mat)
%%%% 计算姿态角速率指令及其导数

iiuav = 4;
ui = ui_vec(:,iiuav);
duihat = duihat_vec(:,iiuav);
d2uihat = d2uihat_vec(:,iiuav);
Rci = Rci_mat(:,:,iiuav);

ee1 = [1;0;0];
ee2 = [0;1;0];
ee3 = [0;0;1];
RciE3 = ui / norm(ui,2);
PiMat = eye(3,3) - ee3*(ee3');
dRciE3 = (1 / norm(ui,2))*Rci*PiMat*(Rci')*duihat;
Themat = [-RciE3(2)/(1+RciE3(3)),         -RciE3(1)/(1+RciE3(3)),       (RciE3(1)*RciE3(2))/((1+RciE3(3))^2); ...
                   2*RciE3(1)/(1+RciE3(3)),                0,                               1 - (RciE3(1)^2)/((1+RciE3(3))^2); ...
                               0                                       -1                                                        0                                   ];
wcxe3 = (1 / norm(ui,2))*PiMat*(Rci')*duihat;
wcxe2 = (1 / norm(ui,2))*(Rci')*Themat*Rci*PiMat*(Rci')*duihat;
wci = [-wcxe3(2); wcxe3(1); -wcxe2(1)];

TempMat1 = [0,                           -1/(1+RciE3(3)),                   (RciE3(2))/((1+RciE3(3))^2); ...
                       2/(1+RciE3(3)),                0,                               (-2*RciE3(1))/((1+RciE3(3))^2); ...
                       0,                                     0,                                                   0                             ];
TempMat2 = [-1/(1+RciE3(3)),              0,                               (RciE3(1))/((1+RciE3(3))^2); ...
                       0,                                     0,                                                   0                      ; ...
                       0,                                     0,                                                   0                             ];
TempMat3 = [(RciE3(2))/((1+RciE3(3))^2),                 (RciE3(1))/((1+RciE3(3))^2),       (-2*RciE3(1)*RciE3(2))/((1+RciE3(3))^3); ...
                       (-2*RciE3(1))/((1+RciE3(3))^2),                             0,                               (2*(RciE3(1)^2))/((1+RciE3(3))^3); ...
                        0,                                                                          0,                                                   0                             ];
dTheMat = TempMat1*dRciE3*(ee1') + TempMat2*dRciE3*(ee2') + TempMat3*dRciE3*(ee3');
wcix = cal_askew_mat(wci);
dRciT = -wcix*(Rci');
dwcxe3 = (1 / norm(ui,2))*PiMat*(dRciT*duihat+(Rci')*(d2uihat-(((ui')*duihat)/(norm(ui,2)^2))*duihat));
dwcxe2 = (1 / norm(ui,2))*((dRciT*Themat+(Rci')*dTheMat) ...
                *(Rci*PiMat*(Rci'))*duihat + (Rci')*Themat*(Rci*PiMat*(Rci'))*(d2uihat-(((ui')*duihat)/(norm(ui,2)^2))*duihat));
dwci = [-dwcxe3(2);  dwcxe3(1);  -dwcxe2(1)];
